simulink library "PAYLOAD_MASTER"  (Simulink 8.8)
settings: Solver=ode45  StartTime=0.0  StopTime=10.0  RelTol=1e-3  EnableMultiTasking=on
libraries: cdsEpicsOut x123, cdsFilt x55, cdsTP x42, cdsFiltCtrl x33, cdsEpicsIn x31, cdsMuxMatrix x17, cdsEpicsBinIn x17, VIS_LIB x13, PAYLOAD_MASTER x13, cdsRms x8, simulink x6, cdsEpicsStringIn x6
(part 2 of 12)

== system PAYLOAD_MASTER/PAYLOADOPLEV ==
  SEG1_in : Inport
  SEG2_in : Inport  Port=2
  SEG3_in : Inport  Port=3
  SEG4_in : Inport  Port=4
  AWHITEN_SET1 : cdsEpicsBinIn/Subsystem  Tag=cdsEpicsBinIn  Description=|
      | Purpose:                                                                            
      | Create an EPICS binary (0 or 1) input channel to the FE realtime controls.          
      |                                                                                     
      | Operation:                                                                          
      | Outputs value from an EPICS ai record. Value is binary input (bi Epics record type).
      |                                                                                     
      | Usage:                                                                              
      | Name the part with the desired EPICS channel name.
      settings: AttributesFormatString=%<Tag>
  AWHITEN_SET2 : cdsEpicsBinIn/Subsystem  Tag=cdsEpicsBinIn  Description=|
      | Purpose:                                                                            
      | Create an EPICS binary (0 or 1) input channel to the FE realtime controls.          
      |                                                                                     
      | Operation:                                                                          
      | Outputs value from an EPICS ai record. Value is binary input (bi Epics record type).
      |                                                                                     
      | Usage:                                                                              
      | Name the part with the desired EPICS channel name.
      settings: AttributesFormatString=%<Tag>
  AWHITEN_SET3 : cdsEpicsBinIn/Subsystem  Tag=cdsEpicsBinIn  Description=|
      | Purpose:                                                                            
      | Create an EPICS binary (0 or 1) input channel to the FE realtime controls.          
      |                                                                                     
      | Operation:                                                                          
      | Outputs value from an EPICS ai record. Value is binary input (bi Epics record type).
      |                                                                                     
      | Usage:                                                                              
      | Name the part with the desired EPICS channel name.
      settings: AttributesFormatString=%<Tag>
  CRS : cdsFilt/Subsystem  Tag=cdsFilt  Description=|
      | Purpose:                                                                                                                                                                                                                                  
      | Standard CDS IIR filter module.                                                                                                                                                                                                           
      |                                                                                                                                                                                                                                           
      | Operation:                                                                                                                                                                                                                                
      | Consists of 10 second order section IIR filters, plus a ramped gain stage. In FE code, also provides pre-defined test points and excitation channel inputs. The filter coefficients are defined in the LIGO system using the 'foton' tool.
      |                                                                                                                                                                                                                                           
      | Usage:                                                                                                                                                                                                                                    
      | Name the part with the desired filter module name.
      settings: AttributesFormatString=%<Tag>
  Constant : Constant  Value=7
  Demux : Demux
  Ground{1..4} (4 alike) : Ground
  MTRX : cdsMuxMatrix/Subsystem  Tag=cdsMuxMatrix  Description=Any size matrix. Inputs and outputs must be connected using Mux and Demux parts.
      settings: AttributesFormatString=%<Tag>
  MTRX_P_OUTMON : cdsEpicsOut/Subsystem  Tag=cdsEpicsOutput  Description=|
      | Purpose:                                          
      | Output a FE signal to an EPICS channel.           
      |                                                   
      | Operation:                                        
      | Takes input value and passes it to EPICS record.  
      |                                                   
      | Usage:                                            
      | Name the part with the desired EPICS rrecord name.
      settings: AttributesFormatString=%<Tag>
  MTRX_Y_OUTMON : cdsEpicsOut/Subsystem  Tag=cdsEpicsOutput  Description=|
      | Purpose:                                          
      | Output a FE signal to an EPICS channel.           
      |                                                   
      | Operation:                                        
      | Takes input value and passes it to EPICS record.  
      |                                                   
      | Usage:                                            
      | Name the part with the desired EPICS rrecord name.
      settings: AttributesFormatString=%<Tag>
  Mux : Mux
  PIT : cdsFilt/Subsystem  Tag=cdsFilt  Description=|
      | Purpose:                                                                                                                                                                                                                                  
      | Standard CDS IIR filter module.                                                                                                                                                                                                           
      |                                                                                                                                                                                                                                           
      | Operation:                                                                                                                                                                                                                                
      | Consists of 10 second order section IIR filters, plus a ramped gain stage. In FE code, also provides pre-defined test points and excitation channel inputs. The filter coefficients are defined in the LIGO system using the 'foton' tool.
      |                                                                                                                                                                                                                                           
      | Usage:                                                                                                                                                                                                                                    
      | Name the part with the desired filter module name.
      settings: AttributesFormatString=%<Tag>
  PIT_NORM : Product  Inputs=*/
  SEG1 : cdsFiltCtrl/IIR FM with control  Tag=cdsFiltCtrl  Description=|
      | cdsFiltCntrl is the standard IIR filter module (exactly the same as cdsFilt) but with added control data output 'Ctrl'. Filter module digital signal output appears on the first output, which is called 'Val'. 'Ctrl' output has a bit pattern encoding the state of filter's on/off switches (FM1 through FM10). The bit values are:
      |                                                                                                                                                                                                                                                                                                                                       
      | module 	hex	dec                                                                                                                                                                                                                                                                                                                       
      | -----------------------                                                                                                                                                                                                                                                                                                               
      | FM1	0x20                    32                                                                                                                                                                                                                                                                                                        
      | FM2	0x80                     128                                                                                                                                                                                                                                                                                                      
      | FM3	0x200                   512                                                                                                                                                                                                                                                                                                       
      | FM4	0x800                   2048                                                                                                                                                                                                                                                                                                      
      | FM5	0x2000                 8192                                                                                                                                                                                                                                                                                                       
      | FM6	0x8000                 32768                                                                                                                                                                                                                                                                                                      
      | FM7	0x20000                131072                                                                                                                                                                                                                                                                                                     
      | FM8	0x80000                 524288                                                                                                                                                                                                                                                                                                    
      | FM9	0x200000               2097152                                                                                                                                                                                                                                                                                                    
      | FM10	0x800000               8388608                                                                                                                                                                                                                                                                                                   
      |                                                                                                                                                                                                                                                                                                                                       
      | This bit data can be used to drive some other switches or it can be output using a binary I/O module.
      settings: AttributesFormatString=%<Tag>
  SEG2 : cdsFiltCtrl/IIR FM with control  Tag=cdsFiltCtrl  Description=|
      | cdsFiltCntrl is the standard IIR filter module (exactly the same as cdsFilt) but with added control data output 'Ctrl'. Filter module digital signal output appears on the first output, which is called 'Val'. 'Ctrl' output has a bit pattern encoding the state of filter's on/off switches (FM1 through FM10). The bit values are:
      |                                                                                                                                                                                                                                                                                                                                       
      | module 	hex	dec                                                                                                                                                                                                                                                                                                                       
      | -----------------------                                                                                                                                                                                                                                                                                                               
      | FM1	0x20                    32                                                                                                                                                                                                                                                                                                        
      | FM2	0x80                     128                                                                                                                                                                                                                                                                                                      
      | FM3	0x200                   512                                                                                                                                                                                                                                                                                                       
      | FM4	0x800                   2048                                                                                                                                                                                                                                                                                                      
      | FM5	0x2000                 8192                                                                                                                                                                                                                                                                                                       
      | FM6	0x8000                 32768                                                                                                                                                                                                                                                                                                      
      | FM7	0x20000                131072                                                                                                                                                                                                                                                                                                     
      | FM8	0x80000                 524288                                                                                                                                                                                                                                                                                                    
      | FM9	0x200000               2097152                                                                                                                                                                                                                                                                                                    
      | FM10	0x800000               8388608                                                                                                                                                                                                                                                                                                   
      |                                                                                                                                                                                                                                                                                                                                       
      | This bit data can be used to drive some other switches or it can be output using a binary I/O module.
      settings: AttributesFormatString=%<Tag>
  SEG3 : cdsFiltCtrl/IIR FM with control  Tag=cdsFiltCtrl  Description=|
      | cdsFiltCntrl is the standard IIR filter module (exactly the same as cdsFilt) but with added control data output 'Ctrl'. Filter module digital signal output appears on the first output, which is called 'Val'. 'Ctrl' output has a bit pattern encoding the state of filter's on/off switches (FM1 through FM10). The bit values are:
      |                                                                                                                                                                                                                                                                                                                                       
      | module 	hex	dec                                                                                                                                                                                                                                                                                                                       
      | -----------------------                                                                                                                                                                                                                                                                                                               
      | FM1	0x20                    32                                                                                                                                                                                                                                                                                                        
      | FM2	0x80                     128                                                                                                                                                                                                                                                                                                      
      | FM3	0x200                   512                                                                                                                                                                                                                                                                                                       
      | FM4	0x800                   2048                                                                                                                                                                                                                                                                                                      
      | FM5	0x2000                 8192                                                                                                                                                                                                                                                                                                       
      | FM6	0x8000                 32768                                                                                                                                                                                                                                                                                                      
      | FM7	0x20000                131072                                                                                                                                                                                                                                                                                                     
      | FM8	0x80000                 524288                                                                                                                                                                                                                                                                                                    
      | FM9	0x200000               2097152                                                                                                                                                                                                                                                                                                    
      | FM10	0x800000               8388608                                                                                                                                                                                                                                                                                                   
      |                                                                                                                                                                                                                                                                                                                                       
      | This bit data can be used to drive some other switches or it can be output using a binary I/O module.
      settings: AttributesFormatString=%<Tag>
  SEG4 : cdsFiltCtrl/IIR FM with control  Tag=cdsFiltCtrl  Description=|
      | cdsFiltCntrl is the standard IIR filter module (exactly the same as cdsFilt) but with added control data output 'Ctrl'. Filter module digital signal output appears on the first output, which is called 'Val'. 'Ctrl' output has a bit pattern encoding the state of filter's on/off switches (FM1 through FM10). The bit values are:
      |                                                                                                                                                                                                                                                                                                                                       
      | module 	hex	dec                                                                                                                                                                                                                                                                                                                       
      | -----------------------                                                                                                                                                                                                                                                                                                               
      | FM1	0x20                    32                                                                                                                                                                                                                                                                                                        
      | FM2	0x80                     128                                                                                                                                                                                                                                                                                                      
      | FM3	0x200                   512                                                                                                                                                                                                                                                                                                       
      | FM4	0x800                   2048                                                                                                                                                                                                                                                                                                      
      | FM5	0x2000                 8192                                                                                                                                                                                                                                                                                                       
      | FM6	0x8000                 32768                                                                                                                                                                                                                                                                                                      
      | FM7	0x20000                131072                                                                                                                                                                                                                                                                                                     
      | FM8	0x80000                 524288                                                                                                                                                                                                                                                                                                    
      | FM9	0x200000               2097152                                                                                                                                                                                                                                                                                                    
      | FM10	0x800000               8388608                                                                                                                                                                                                                                                                                                   
      |                                                                                                                                                                                                                                                                                                                                       
      | This bit data can be used to drive some other switches or it can be output using a binary I/O module.
      settings: AttributesFormatString=%<Tag>
  SUM : cdsFilt/Subsystem  Tag=cdsFilt  Description=|
      | Purpose:                                                                                                                                                                                                                                  
      | Standard CDS IIR filter module.                                                                                                                                                                                                           
      |                                                                                                                                                                                                                                           
      | Operation:                                                                                                                                                                                                                                
      | Consists of 10 second order section IIR filters, plus a ramped gain stage. In FE code, also provides pre-defined test points and excitation channel inputs. The filter coefficients are defined in the LIGO system using the 'foton' tool.
      |                                                                                                                                                                                                                                           
      | Usage:                                                                                                                                                                                                                                    
      | Name the part with the desired filter module name.
      settings: AttributesFormatString=%<Tag>
  Saturation : Saturate  UpperLimit=1e12  LowerLimit=1
  YAW : cdsFilt/Subsystem  Tag=cdsFilt  Description=|
      | Purpose:                                                                                                                                                                                                                                  
      | Standard CDS IIR filter module.                                                                                                                                                                                                           
      |                                                                                                                                                                                                                                           
      | Operation:                                                                                                                                                                                                                                
      | Consists of 10 second order section IIR filters, plus a ramped gain stage. In FE code, also provides pre-defined test points and excitation channel inputs. The filter coefficients are defined in the LIGO system using the 'foton' tool.
      |                                                                                                                                                                                                                                           
      | Usage:                                                                                                                                                                                                                                    
      | Name the part with the desired filter module name.
      settings: AttributesFormatString=%<Tag>
  YAW_NORM : Product  Inputs=*/
  cdsBit2Word : cdsBit2Word/cdsBit2Word  Tag=cdsBit2Word  Description=Forms single 16 bit integer from 16 0/1 inputs.
      settings: AttributesFormatString=%<Tag>
  PIT_out : Outport
  YAW_out : Outport  Port=2
  SUM_out : Outport  Port=3
  CRS_Out : Outport  Port=4
  WHT_CTRL_SEG1 : Outport  Port=5
  WHT_CTRL_SEG2 : Outport  Port=6
  WHT_CTRL_SEG3 : Outport  Port=7
  WHT_CTRL_SEG4 : Outport  Port=8
  wires:
  cdsBit2Word/1 -> SEG4/2, SEG3/2, SEG2/2, SEG1/2
  Constant/1 -> SEG4/3, SEG3/3, SEG2/3, SEG1/3
  Ground4/1 -> cdsBit2Word/4, cdsBit2Word/5, cdsBit2Word/6, cdsBit2Word/7, cdsBit2Word/8, cdsBit2Word/9, cdsBit2Word/10, cdsBit2Word/11, cdsBit2Word/12, cdsBit2Word/13, cdsBit2Word/14, cdsBit2Word/15, cdsBit2Word/16
  AWHITEN_SET3/1 -> cdsBit2Word/3
  AWHITEN_SET2/1 -> cdsBit2Word/2
  AWHITEN_SET1/1 -> cdsBit2Word/1
  Ground3/1 -> AWHITEN_SET3/1
  Ground2/1 -> AWHITEN_SET2/1
  Ground1/1 -> AWHITEN_SET1/1
  SEG1_in/1 -> SEG1/1
  SEG2_in/1 -> SEG2/1
  SEG3_in/1 -> SEG3/1
  SEG4_in/1 -> SEG4/1
  Mux/1 -> MTRX/1
  MTRX/1 -> Demux/1
  SEG1/1 -> Mux/1
  SEG2/1 -> Mux/2
  SEG3/1 -> Mux/3
  SEG4/1 -> Mux/4
  PIT/1 -> PIT_out/1
  YAW/1 -> YAW_out/1
  SUM/1 -> Saturation/1, SUM_out/1
  PIT_NORM/1 -> PIT/1
  YAW_NORM/1 -> YAW/1
  Demux/1 -> MTRX_P_OUTMON/1
  Demux/3 -> SUM/1
  Demux/2 -> MTRX_Y_OUTMON/1
  Saturation/1 -> YAW_NORM/2, PIT_NORM/2
  MTRX_P_OUTMON/1 -> PIT_NORM/1
  MTRX_Y_OUTMON/1 -> YAW_NORM/1
  Demux/4 -> CRS/1
  CRS/1 -> CRS_Out/1
  SEG1/2 -> WHT_CTRL_SEG1/1
  SEG2/2 -> WHT_CTRL_SEG2/1
  SEG3/2 -> WHT_CTRL_SEG3/1
  SEG4/2 -> WHT_CTRL_SEG4/1

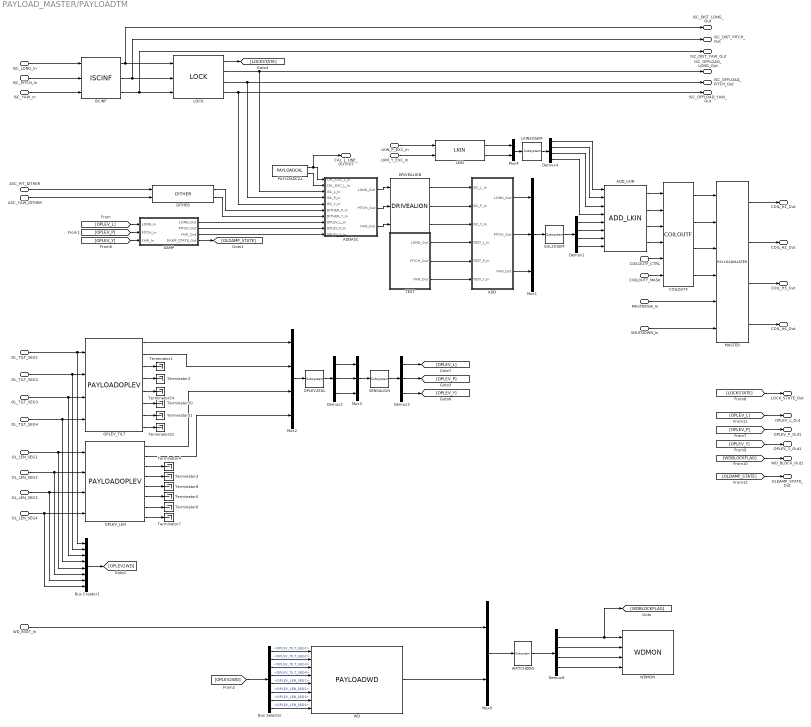
== system PAYLOAD_MASTER/PAYLOADTM ==
  ISC_LONG_In : Inport
  ISC_PITCH_In : Inport  Port=2
  ISC_YAW_In : Inport  Port=3
  COILOUTF_CTRL : Inport  Port=4
  COILOUTF_MASK : Inport  Port=5
  OL_TILT_SEG1 : Inport  Port=6
  OL_TILT_SEG2 : Inport  Port=7
  OL_TILT_SEG3 : Inport  Port=8
  OL_TILT_SEG4 : Inport  Port=9
  OL_LEN_SEG1 : Inport  Port=10
  OL_LEN_SEG2 : Inport  Port=11
  OL_LEN_SEG3 : Inport  Port=12
  OL_LEN_SEG4 : Inport  Port=13
  MASTERSW_In : Inport  Port=14
  ASC_PIT_DITHER : Inport  Port=15
  ASC_YAW_DITHER : Inport  Port=16
  LKIN_P_EXC_In : Inport  Port=17
  LKIN_Y_EXC_In : Inport  Port=18
  WD_RSET_In : Inport  Port=19
  SHUTDOWN_In : Inport  Port=20
  ADD : Subsystem
  ADDASC : Subsystem
  ADD_LKIN : VIS_LIB/ADD_LKIN
  Bus Creator1 : BusCreator  Inputs='OPLEV_TILT_SEG1','OPLEV_TILT_SEG2','OPLEV_TILT_SEG3','OPLEV_TILT_SEG4','OPLEV_LEN_SEG1','OPLEV_LEN_SEG2','OPLEV_LEN_SEG3','OPLEV_LEN_SEG4'
  Bus Selector : BusSelector  OutputSignals=OPLEV_TILT_SEG1,OPLEV_TILT_SEG2,OPLEV_TILT_SEG3,OPLEV_TILT_SEG4,OPLEV_LEN_SEG1,OPLEV_LEN_SEG2,OPLEV_LEN_SEG3,OPLEV_LEN_SEG4
  COILOUTF : FOUROSEM_COILOUTF_MASTER/COILOUTF
  DAMP : Subsystem
  DITHER : VIS_LIB/DITHER
  DRIVEALIGN : VIS_LIB/DRIVEALIGN
  Demux1 : Demux
  Demux2 : Demux  Outputs=3
  Demux3 : Demux  Outputs=3
  Demux4 : Demux
  Demux9 : Demux
  EUL2OSEM : cdsMuxMatrix/Subsystem  Tag=cdsMuxMatrix  Description=Any size matrix. Inputs and outputs must be connected using Mux and Demux parts.
      settings: AttributesFormatString=%<Tag>
  ISCINF : VIS_LIB/ISCINF
  LKIN : VIS_LIB/LKIN
  LKIN2OSEM : cdsMuxMatrix/Subsystem  Tag=cdsMuxMatrix  Description=Any size matrix. Inputs and outputs must be connected using Mux and Demux parts.
      settings: AttributesFormatString=%<Tag>
  LOCK : VIS_LIB/LOCK
  MASTER : PAYLOAD_MASTER/PAYLOADMASTER
  Mux1 : Mux  Inputs=3
  Mux2 : Mux
  Mux3 : Mux  Inputs=3
  Mux4 : Mux  Inputs=2
  Mux9 : Mux  Inputs=2
  OPLEV2EUL : cdsMuxMatrix/Subsystem  Tag=cdsMuxMatrix  Description=Any size matrix. Inputs and outputs must be connected using Mux and Demux parts.
      settings: AttributesFormatString=%<Tag>
  OPLEV_LEN : PAYLOAD_MASTER/PAYLOADOPLEV
  OPLEV_TILT : PAYLOAD_MASTER/PAYLOADOPLEV
  PAYLOADCAL : PAYLOAD_MASTER/PAYLOADCAL
  SENSALIGN : cdsMuxMatrix/Subsystem  Tag=cdsMuxMatrix  Description=Any size matrix. Inputs and outputs must be connected using Mux and Demux parts.
      settings: AttributesFormatString=%<Tag>
  TEST : Subsystem
  Terminator{1..8,50..52,54} (12 alike) : Terminator
  WATCHDOG : cdsFunctionCall/Subsystem  Tag=cdsFunctionCall  Description=inline OSEMWATCHDOG /opt/rtcds/userapps/release/vis/common/src/WATCHDOG.c
      settings: AttributesFormatString=%<Tag>\n%<Description>
  WD : PAYLOAD_MASTER/PAYLOADWD
  WDMON : PAYLOAD_MASTER/PAYLOADIM/WDMON
  COIL_H1_Out : Outport
  COIL_H2_Out : Outport  Port=2
  COIL_H3_Out : Outport  Port=3
  COIL_H4_Out : Outport  Port=4
  LOCK_STATE_Out : Outport  Port=5
  ISC_DIST_LONG_Out : Outport  Port=6
  ISC_DIST_PITCH_Out : Outport  Port=7
  ISC_DIST_YAW_Out : Outport  Port=8
  ISC_OFFLOAD_LONG_Out : Outport  Port=9
  ISC_OFFLOAD_PITCH_Out : Outport  Port=10
  ISC_OFFLOAD_YAW_Out : Outport  Port=11
  CAL_L_LINE_OUTPUT : Outport  Port=12
  OPLEV_L_Out : Outport  Port=13
  OPLEV_P_Out1 : Outport  Port=14
  OPLEV_Y_Out1 : Outport  Port=15
  WD_BLOCK_Out1 : Outport  Port=16
  OLDAMP_STATE_Out : Outport  Port=17
  wires:
  ISC_PITCH_In/1 -> ISCINF/2
  ISC_LONG_In/1 -> ISCINF/1
  ISC_YAW_In/1 -> ISCINF/3
  LKIN_Y_EXC_In/1 -> LKIN/2
  LKIN_P_EXC_In/1 -> LKIN/1
  LOCK/1 -> [LOCKSTATE]
  [LOCKSTATE] -> LOCK_STATE_Out/1
  MASTERSW_In/1 -> MASTER/5
  ADD_LKIN/4 -> COILOUTF/4
  ADD_LKIN/3 -> COILOUTF/3
  ADD_LKIN/2 -> COILOUTF/2
  ADD_LKIN/1 -> COILOUTF/1
  Demux1/4 -> ADD_LKIN/8
  Demux1/3 -> ADD_LKIN/7
  Demux1/2 -> ADD_LKIN/6
  Demux1/1 -> ADD_LKIN/5
  Demux4/4 -> ADD_LKIN/4
  Demux4/3 -> ADD_LKIN/3
  Demux4/2 -> ADD_LKIN/2
  LKIN/2 -> Mux4/2
  LKIN/1 -> Mux4/1
  Demux4/1 -> ADD_LKIN/1
  LKIN2OSEM/1 -> Demux4/1
  Mux4/1 -> LKIN2OSEM/1
  MASTER/4 -> COIL_H4_Out/1
  MASTER/3 -> COIL_H3_Out/1
  MASTER/2 -> COIL_H2_Out/1
  MASTER/1 -> COIL_H1_Out/1
  DRIVEALIGN/3 -> ADD/3(ISC_Y_In)
  DRIVEALIGN/2 -> ADD/2(ISC_P_In)
  DRIVEALIGN/1 -> ADD/1(ISC_L_In)
  ADDASC/3(YAW_Out) -> DRIVEALIGN/3
  ADDASC/2(PITCH_Out) -> DRIVEALIGN/2
  ADD/1(LONG_Out) -> Mux1/1
  ADD/2(PITCH_Out) -> Mux1/2
  ADD/3(YAW_Out) -> Mux1/3
  DITHER/2 -> ADDASC/7(DITHER_Y_In)
  DITHER/1 -> ADDASC/6(DITHER_P_In)
  ASC_YAW_DITHER/1 -> DITHER/2
  ASC_PIT_DITHER/1 -> DITHER/1
  Mux1/1 -> EUL2OSEM/1
  EUL2OSEM/1 -> Demux1/1
  COILOUTF/1 -> MASTER/1
  COILOUTF/2 -> MASTER/2
  COILOUTF/3 -> MASTER/3
  COILOUTF/4 -> MASTER/4
  COILOUTF_MASK/1 -> COILOUTF/6
  COILOUTF_CTRL/1 -> COILOUTF/5
  TEST/1(LONG_Out) -> ADD/4(TEST_L_In)
  TEST/2(PITCH_Out) -> ADD/5(TEST_P_In)
  TEST/3(YAW_Out) -> ADD/6(TEST_Y_In)
  ISCINF/1 -> ISC_DIST_LONG_Out/1, LOCK/1
  ISCINF/2 -> ISC_DIST_PITCH_Out/1, LOCK/2
  ISCINF/3 -> ISC_DIST_YAW_Out/1, LOCK/3
  SHUTDOWN_In/1 -> MASTER/6
  LOCK/2 -> ADDASC/3(ISC_L_In), ISC_OFFLOAD_LONG_Out/1
  LOCK/3 -> ADDASC/4(ISC_P_In), ISC_OFFLOAD_PITCH_Out/1
  LOCK/4 -> ADDASC/5(ISC_Y_In), ISC_OFFLOAD_YAW_Out/1
  OPLEV_TILT/6 -> Terminator50/1
  OPLEV_TILT/8 -> Terminator52/1
  OPLEV_TILT/7 -> Terminator51/1
  OPLEV_TILT/5 -> Terminator54/1
  OPLEV_LEN/8 -> Terminator7/1
  OPLEV_LEN/7 -> Terminator6/1
  OPLEV_LEN/6 -> Terminator5/1
  OPLEV_LEN/5 -> Terminator8/1
  OL_TILT_SEG1/1 -> OPLEV_TILT/1, Bus Creator1/1
  OL_TILT_SEG2/1 -> OPLEV_TILT/2, Bus Creator1/2
  OL_TILT_SEG3/1 -> OPLEV_TILT/3, Bus Creator1/3
  OL_TILT_SEG4/1 -> OPLEV_TILT/4, Bus Creator1/4
  OL_LEN_SEG1/1 -> OPLEV_LEN/1, Bus Creator1/5
  OL_LEN_SEG2/1 -> OPLEV_LEN/2, Bus Creator1/6
  OL_LEN_SEG3/1 -> OPLEV_LEN/3, Bus Creator1/7
  OL_LEN_SEG4/1 -> OPLEV_LEN/4, Bus Creator1/8
  Mux2/1 -> OPLEV2EUL/1
  OPLEV2EUL/1 -> Demux2/1
  Mux3/1 -> SENSALIGN/1
  SENSALIGN/1 -> Demux3/1
  Demux2/1 -> Mux3/1
  Demux2/2 -> Mux3/2
  Demux2/3 -> Mux3/3
  Demux3/2 -> [OPLEV_P]
  Demux3/3 -> [OPLEV_Y]
  WD_RSET_In/1 -> Mux9/1
  WD/1 -> Mux9/2
  [OPLEV2WD] -> Bus Selector/1
  Demux9/1 -> WDMON/1, [WDBLOCKFLAG]
  Demux9/2 -> WDMON/2
  Demux9/3 -> WDMON/3
  Demux9/4 -> WDMON/4
  Mux9/1 -> WATCHDOG/1
  WATCHDOG/1 -> Demux9/1
  Bus Creator1/1 -> [OPLEV2WD]
  Bus Selector/1 -> WD/1  "<OPLEV_TILT_SEG1>"
  Bus Selector/2 -> WD/2  "<OPLEV_TILT_SEG2>"
  Bus Selector/3 -> WD/3  "<OPLEV_TILT_SEG3>"
  Bus Selector/4 -> WD/4  "<OPLEV_TILT_SEG4>"
  Bus Selector/5 -> WD/5  "<OPLEV_LEN_SEG1>"
  Bus Selector/6 -> WD/6  "<OPLEV_LEN_SEG2>"
  Bus Selector/7 -> WD/7  "<OPLEV_LEN_SEG3>"
  Bus Selector/8 -> WD/8  "<OPLEV_LEN_SEG4>"
  ADDASC/1(LONG_Out) -> DRIVEALIGN/1
  PAYLOADCAL/2 -> ADDASC/2(CAL_EXC_L_In)
  PAYLOADCAL/1 -> ADDASC/1(CAL_OSC_L_In), CAL_L_LINE_OUTPUT/1
  OPLEV_TILT/1 -> Mux2/1
  OPLEV_TILT/2 -> Mux2/2
  OPLEV_LEN/1 -> Mux2/3
  OPLEV_LEN/2 -> Mux2/4
  OPLEV_TILT/4 -> Terminator2/1
  OPLEV_TILT/3 -> Terminator1/1
  OPLEV_LEN/3 -> Terminator4/1
  OPLEV_LEN/4 -> Terminator3/1
  [OPLEV_L] -> DAMP/1(LONG_In)
  [OPLEV_P] -> DAMP/2(PITCH_In)
  [OPLEV_Y] -> DAMP/3(YAW_In)
  DAMP/1(LONG_Out) -> ADDASC/8(OPLEV_L_In)
  DAMP/2(PITCH_Out) -> ADDASC/9(OPLEV_P_In)
  DAMP/3(YAW_Out) -> ADDASC/10(OPLEV_Y_In)
  DAMP/4(DAMP_STATE_Out) -> [OLDAMP_STATE]
  [OPLEV_P] -> OPLEV_P_Out1/1
  [OPLEV_Y] -> OPLEV_Y_Out1/1
  [WDBLOCKFLAG] -> WD_BLOCK_Out1/1
  [OPLEV_L] -> OPLEV_L_Out/1
  [OLDAMP_STATE] -> OLDAMP_STATE_Out/1
  Demux3/1 -> [OPLEV_L]

== system PAYLOAD_MASTER/PAYLOADWD ==
  OPLEV_TILT_SEG1_In : Inport
  OPLEV_TILT_SEG2_In : Inport  Port=2
  OPLEV_TILT_SEG3_In : Inport  Port=3
  OPLEV_TILT_SEG4_In : Inport  Port=4
  OPLEV_LEN_SEG1_In : Inport  Port=5
  OPLEV_LEN_SEG2_In : Inport  Port=6
  OPLEV_LEN_SEG3_In : Inport  Port=7
  OPLEV_LEN_SEG4_In : Inport  Port=8
  OPLEVAC : Subsystem
  OPLEV_AC_FLAG_Out : Outport
  wires:
  OPLEV_TILT_SEG1_In/1 -> OPLEVAC/1(TILT_SEG1_In)
  OPLEVAC/1(FLAG) -> OPLEV_AC_FLAG_Out/1
  OPLEV_TILT_SEG2_In/1 -> OPLEVAC/2(TILT_SEG2_In)
  OPLEV_TILT_SEG3_In/1 -> OPLEVAC/3(TILT_SEG3_In)
  OPLEV_TILT_SEG4_In/1 -> OPLEVAC/4(TILT_SEG4_In)
  OPLEV_LEN_SEG1_In/1 -> OPLEVAC/5(LEN_SEG1_In)
  OPLEV_LEN_SEG2_In/1 -> OPLEVAC/6(LEN_SEG2_In)
  OPLEV_LEN_SEG3_In/1 -> OPLEVAC/7(LEN_SEG3_In)
  OPLEV_LEN_SEG4_In/1 -> OPLEVAC/8(LEN_SEG4_In)
